simulink model "Quartercar_model"  (R2024b)
settings: Solver=VariableStepAuto  StartTime=0.0  StopTime=30  RelTol=1e-3
settings Model: Creator=kanishka  LastModifiedBy=kanishka

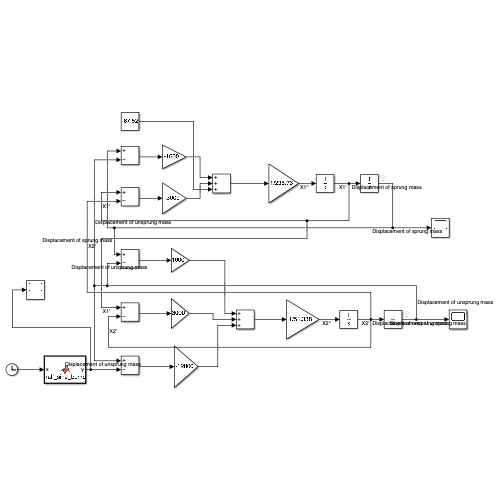
[thumbnail: Simulink's stored preview of the top-level diagram]
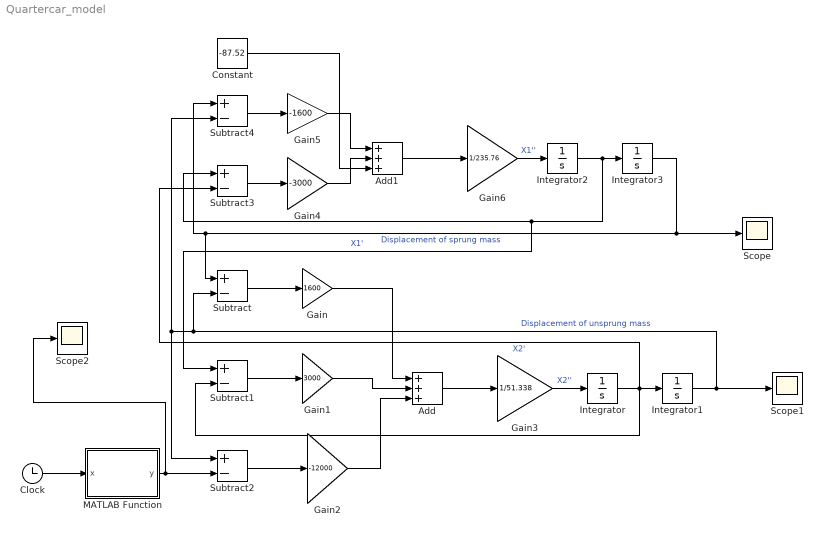
== system Quartercar_model ==
  Add : Sum  Inputs=+++
  Add1 : Sum  Inputs=+++
  Clock : Clock
  Constant : Constant  Value=-87.52
  Gain : Gain  Gain=1600
  Gain1 : Gain  Gain=3000
  Gain2 : Gain  Gain=-12000
  Gain3 : Gain  Gain=1/51.338
  Gain4 : Gain  Gain=-3000
  Gain5 : Gain  Gain=-1600
  Gain6 : Gain  Gain=1/235.76
  Integrator{,1..3} (4 alike) : Integrator
  MATLAB Function : MATLAB Function  TreatAsAtomicUnit=on
  Scope : Scope
  Scope1 : Scope
  Scope2 : Scope
  Subtract{,1..4} (5 alike) : Sum  Inputs=+-
  wires:
  Subtract1/1 -> Gain1/1
  Subtract/1 -> Gain/1
  Subtract2/1 -> Gain2/1
  Gain/1 -> Add/1
  Gain1/1 -> Add/2
  Gain2/1 -> Add/3
  Add/1 -> Gain3/1
  Integrator/1 -> Subtract3/2, Subtract1/2, Integrator1/1  "X2'"
  Gain3/1 -> Integrator/1  "X2''"
  Integrator1/1 -> Scope1/1, Subtract2/1, Subtract4/2, Subtract/2  "Displacement of unsprung mass"
  Subtract3/1 -> Gain4/1
  Subtract4/1 -> Gain5/1
  Gain5/1 -> Add1/1
  Gain4/1 -> Add1/2
  Add1/1 -> Gain6/1
  Gain6/1 -> Integrator2/1  "X1''"
  Integrator2/1 -> Subtract1/1, Subtract3/1, Integrator3/1  "X1'"
  Integrator3/1 -> Scope/1, Subtract/1, Subtract4/1  "Displacement of sprung mass"
  MATLAB Function/1(y) -> Scope2/1, Subtract2/2
  Clock/1 -> MATLAB Function/1(x)
  Constant/1 -> Add1/3

== matlab function Quartercar_model/MATLAB Function ==
  data: x input; y output
function y = half_sine_bump(x)

amplitude = 0.05;     
wavelength = 0.6;      
                



if x >= 0 && x <= wavelength/2
    y = amplitude * sin((2*pi * x) / wavelength);
else
    y = 0;
end
end
